simulink model "Hinf_MISO_Linear_Z1_PbhPin_sim"  (Simulink 7.8)
settings: Solver=ode15s  StartTime=0.0  StopTime=100000  MaxStep=1  MinStep=1e-9  RelTol=1e-8
values from neighbouring files (symbols this model uses):
  K = minreal(K)    [Hinf_Linear_Z1_Prb.m]    (also in Hinf_Linear_Z1_Pwh.m; Hinf_MIMO_Nonlinear_Z1_PwhPrb.m; Hinf_MISO_Nonlinear_Z1_PbhPin.m; Hinf_MISO_Nonlinear_Z1_PbhWin.m)
  sys = (ss(A,Bs,Cs,Ds))    [Hinf_Linear_Z1_Prb.m]    (also in Hinf_Linear_Z1_Pwh.m; Hinf_MIMO_Nonlinear_Z1_PwhPrb.m; Hinf_MISO_Nonlinear_Z1_PbhPin.m; Hinf_MISO_Nonlinear_Z1_PbhWin.m)
settings Model: Creator=jahansha  LastModifiedBy=matslie
settings DebuggingCC: FcnCallInpInsideContextMsg=Use local settings

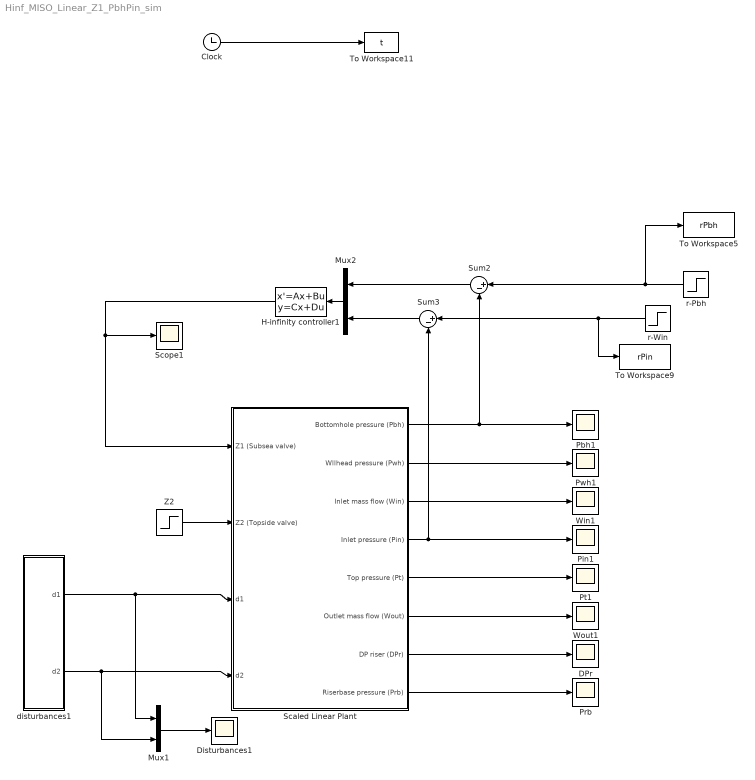
== system Hinf_MISO_Linear_Z1_PbhPin_sim ==
  Clock : Clock
  DPr : Scope
      settings: TimeRange=100000  YMin=-0.6  YMax=1.4
  Disturbances1 : Scope
      settings: TimeRange=8000  YMin=1.38778e-017  YMax=0.275  SaveName=ScopeData8
  H-infinity controller1 : StateSpace  A=K.a  B=K.b  C=K.c  D=K.d
  Mux1 : Mux  Inputs=2
  Mux2 : Mux  Inputs=2
  Pbh1 : Scope
      settings: TimeRange=10000  YMin=-75  YMax=200  SaveName=ScopeData11
  Pin1 : Scope
      settings: TimeRange=8000  YMin=0.105  YMax=0.113  SaveName=ScopeData12
  Prb : Scope
      settings: TimeRange=100000  YMin=-0.6  YMax=1.4
  Pt1 : Scope
      settings: TimeRange=8000  YMin=0.105  YMax=0.113  SaveName=ScopeData13
  Pwh1 : Scope
      settings: TimeRange=10000  YMin=-0.0275  YMax=-0.0075  SaveName=ScopeData14
  Scaled Linear Plant : Subsystem
  Scope1 : Scope
      settings: TimeRange=8000  YMin=-0.4  YMax=1.2  SaveName=ScopeData15
  Sum2 : Sum  Inputs=|+-
  Sum3 : Sum  Inputs=|+-
  To Workspace11 : ToWorkspace  VariableName=t  SampleTime=-1  SaveFormat=Array
  To Workspace5 : ToWorkspace  VariableName=rPbh  SampleTime=-1  SaveFormat=Array
  To Workspace9 : ToWorkspace  VariableName=rPin  SampleTime=-1  SaveFormat=Array
  Win1 : Scope
      settings: YMin=0.225  YMax=0.55  SaveName=ScopeData16
  Wout1 : Scope
      settings: TimeRange=100000  YMin=-0.6  YMax=1.4  SaveName=ScopeData17
  Z2 : Step  Time=0  After=0  SampleTime=0
  disturbances1 : Subsystem
  r-Pbh : Step  Time=100000  After=0  SampleTime=0
  r-Win : Step  Time=10000  After=0  SampleTime=0
  wires:
  Mux1/1 -> Disturbances1/1
  disturbances1/1(d1) -> Mux1/1, Scaled Linear Plant/3(d1)
  disturbances1/2(d2) -> Mux1/2, Scaled Linear Plant/4(d2)
  Scaled Linear Plant/1(Bottomhole pressure (Pbh)) -> Pbh1/1, Sum2/2
  Scaled Linear Plant/2(Wllhead pressure (Pwh)) -> Pwh1/1
  Scaled Linear Plant/3(Inlet mass flow (Win)) -> Win1/1
  Scaled Linear Plant/4(Inlet pressure (Pin)) -> Pin1/1, Sum3/2
  Scaled Linear Plant/5(Top pressure (Pt)) -> Pt1/1
  H-infinity controller1/1 -> Scope1/1, Scaled Linear Plant/1(Z1 (Subsea valve))
  Scaled Linear Plant/6(Outlet mass flow (Wout)) -> Wout1/1
  Z2/1 -> Scaled Linear Plant/2(Z2 (Topside valve))
  Clock/1 -> To Workspace11/1
  r-Pbh/1 -> To Workspace5/1, Sum2/1
  Scaled Linear Plant/7(DP riser (DPr)) -> DPr/1
  Scaled Linear Plant/8(Riserbase pressure (Prb)) -> Prb/1
  Mux2/1 -> H-infinity controller1/1
  Sum2/1 -> Mux2/1
  Sum3/1 -> Mux2/2
  r-Win/1 -> To Workspace9/1, Sum3/1

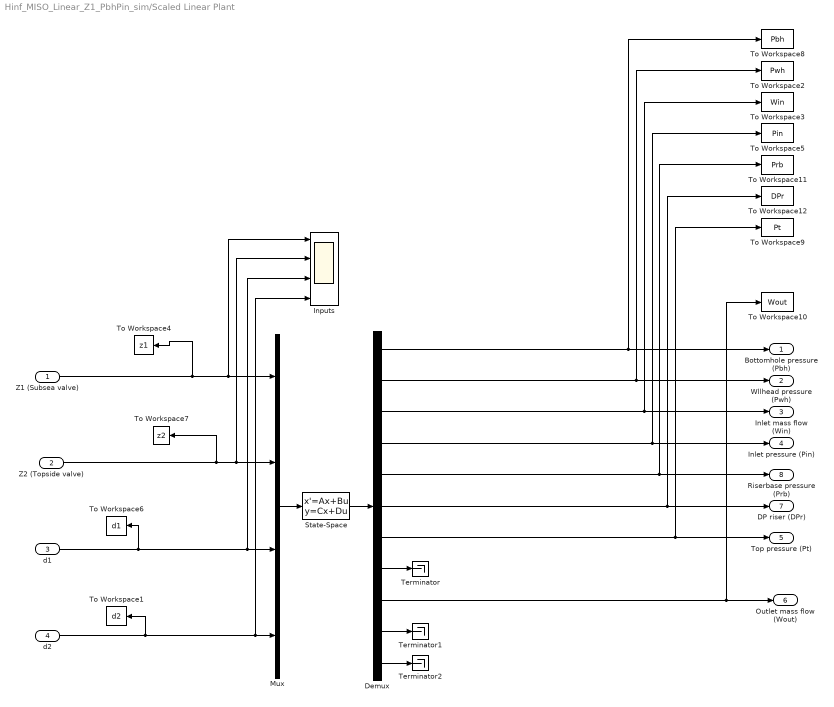
== system Hinf_MISO_Linear_Z1_PbhPin_sim/Scaled Linear Plant ==
  Z1 (Subsea valve) : Inport
  Z2 (Topside valve) : Inport  Port=2
  d1 : Inport  Port=3
  d2 : Inport  Port=4
  Demux : Demux  Outputs=11
  Inputs : Scope  NumInputPorts=4
      settings: TimeRange=8000  YMin=-1~-5~-5~-5  YMax=1~5~5~5  SaveName=ScopeData9
  Mux : Mux
  State-Space : StateSpace  A=sys.a  B=sys.b  C=sys.c  D=sys.d
  Terminator : Terminator
  Terminator1 : Terminator
  Terminator2 : Terminator
  To Workspace1 : ToWorkspace  VariableName=d2  SampleTime=-1  SaveFormat=Array
  To Workspace10 : ToWorkspace  VariableName=Wout  SampleTime=-1  SaveFormat=Array
  To Workspace11 : ToWorkspace  VariableName=Prb  SampleTime=-1  SaveFormat=Array
  To Workspace12 : ToWorkspace  VariableName=DPr  SampleTime=-1  SaveFormat=Array
  To Workspace2 : ToWorkspace  VariableName=Pwh  SampleTime=-1  SaveFormat=Array
  To Workspace3 : ToWorkspace  VariableName=Win  SampleTime=-1  SaveFormat=Array
  To Workspace4 : ToWorkspace  VariableName=z1  SampleTime=-1  SaveFormat=Array
  To Workspace5 : ToWorkspace  VariableName=Pin  SampleTime=-1  SaveFormat=Array
  To Workspace6 : ToWorkspace  VariableName=d1  SampleTime=-1  SaveFormat=Array
  To Workspace7 : ToWorkspace  VariableName=z2  SampleTime=-1  SaveFormat=Array
  To Workspace8 : ToWorkspace  VariableName=Pbh  SampleTime=-1  SaveFormat=Array
  To Workspace9 : ToWorkspace  VariableName=Pt  SampleTime=-1  SaveFormat=Array
  Bottomhole pressure (Pbh) : Outport
  Wllhead pressure (Pwh) : Outport  Port=2
  Inlet mass flow (Win) : Outport  Port=3
  Inlet pressure (Pin) : Outport  Port=4
  Top pressure (Pt) : Outport  Port=5
  Outlet mass flow (Wout) : Outport  Port=6
  DP riser (DPr) : Outport  Port=7
  Riserbase pressure (Prb) : Outport  Port=8
  wires:
  Mux/1 -> State-Space/1
  State-Space/1 -> Demux/1
  Demux/1 -> Bottomhole pressure (Pbh)/1, To Workspace8/1
  Demux/2 -> Wllhead pressure (Pwh)/1, To Workspace2/1
  Demux/3 -> Inlet mass flow (Win)/1, To Workspace3/1
  Demux/4 -> Inlet pressure (Pin)/1, To Workspace5/1
  Z1 (Subsea valve)/1 -> Inputs/1, Mux/1, To Workspace4/1
  d1/1 -> Mux/3, Inputs/3, To Workspace6/1
  d2/1 -> Mux/4, Inputs/4, To Workspace1/1
  Z2 (Topside valve)/1 -> Mux/2, Inputs/2, To Workspace7/1
  Demux/7 -> Top pressure (Pt)/1, To Workspace9/1
  Demux/9 -> Outlet mass flow (Wout)/1, To Workspace10/1
  Demux/6 -> DP riser (DPr)/1, To Workspace12/1
  Demux/5 -> Riserbase pressure (Prb)/1, To Workspace11/1
  Demux/8 -> Terminator/1
  Demux/10 -> Terminator1/1
  Demux/11 -> Terminator2/1

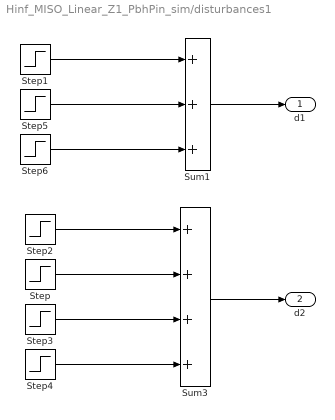
== system Hinf_MISO_Linear_Z1_PbhPin_sim/disturbances1 ==
  Step : Step  Time=30000  After=-1  SampleTime=0
  Step1 : Step  Time=10000  SampleTime=0
  Step2 : Step  Time=20000  SampleTime=0
  Step3 : Step  Time=40000  After=-1  SampleTime=0
  Step4 : Step  Time=60000  SampleTime=0
  Step5 : Step  Time=50000  After=-1  SampleTime=0
  Step6 : Step  Time=70000  After=-1  SampleTime=0
  Sum1 : Sum  Inputs=+++
  Sum3 : Sum  Inputs=++++
  d1 : Outport
  d2 : Outport  Port=2
  wires:
  Sum3/1 -> d2/1
  Sum1/1 -> d1/1
  Step2/1 -> Sum3/1
  Step/1 -> Sum3/2
  Step3/1 -> Sum3/3
  Step4/1 -> Sum3/4
  Step1/1 -> Sum1/1
  Step5/1 -> Sum1/2
  Step6/1 -> Sum1/3
